simulink model "Modelisation_2_MGI_comparaison_avec_Clavel"  (R2015a)
settings: Solver=ode45  StartTime=0.0  StopTime=3  MaxStep=0.001  RelTol=1e-3
undefined symbols (not defined in the file or in its folder): sfun3d
settings Model: Creator=user  LastModifiedBy=user

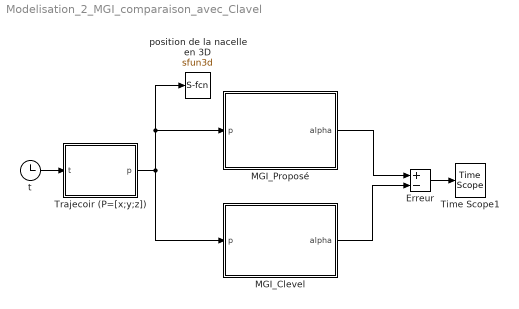
== system Modelisation_2_MGI_comparaison_avec_Clavel ==
  Erreur : Sum  Inputs=+-
  MGI_Clevel : MATLAB Function  TreatAsAtomicUnit=on
  MGI_Proposé : MATLAB Function  TreatAsAtomicUnit=on
  Time Scope1 : TimeScope  DefaultConfigurationName=spbscopes.TimeScopeBlockCfg
  Trajecoir (P=[x;y;z]) : MATLAB Function  TreatAsAtomicUnit=on
  "position de la nacelle en 3D " : S-Function  LoadFcn=sfun3d([],[],[],'LoadBlock')  StartFcn=sfun3d([],[],[],'Start')  StopFcn=sfun3d([],[],[],'Stop')  FunctionName=sfun3d  Parameters=ax,T,np,cp,gd,ls,mk  mask(3D Graph){np=1, ax=[-1 1 -1 1 -2 0]*0.3, cp=[3 2 1], gd=on, ls=-, mk=o, T=0.001}
      mask prompts: np "Number of point (lines)"; ax "[xmin xmax  ymin ymax zmin zmax]"; cp "Camera position (use [0 0 1] for 2D XY view)"; gd "Grid (on|off)"; ls "LineStyle"; mk "Marker"; T "Sampling Time"
      mask help:
      | This block plots the position of several points in the XYZ space. The input contains the coordinates of all the points (x1,y1,z1,x2,y2,z2,...).
      | The number of points (lines), the XYZ ranges, camera position, grid, linestyle, marker and sampling time, can be set as mask parameters.
      settings: CopyFcn=sfun3d([],[],[],'CopyBlock')  DeleteFcn=sfun3d([],[],[],'DeleteBlock')  NameChangeFcn=sfun3d([],[],[],'NameChange')
      mask Help:
      | This block plots the position of several points in the XYZ space. The input contains the coordinates of all the points (x1,y1,z1,x2,y2,z2,...).
      | The number of points (lines), the XYZ ranges, camera position, grid, linestyle, marker and sampling time, can be set as mask parameters.
      mask TypeOptions ls: - | -- | : | -. | none
      mask TypeOptions mk: none | . | + | o | * | x | square | diamond | v | ^ | > | < | pentagram | hexagram
      mask Display: plot([.05 .95 .95 .05 .05],[.45 .45 .95 .95 .45], 0.5+cos(0:0.1:2*pi)*0.3,0.7+sin(0:0.1:2*pi)*0.2)
  t : Clock
  wires:
  t/1 -> Trajecoir (P=[x;y;z])/1(t)
  Erreur/1 -> Time Scope1/1
  Trajecoir (P=[x;y;z])/1(p) -> "position de la nacelle en 3D "/1, MGI_Proposé/1(p), MGI_Clevel/1(p)
  MGI_Proposé/1(alpha) -> Erreur/1
  MGI_Clevel/1(alpha) -> Erreur/2

== matlab function Modelisation_2_MGI_comparaison_avec_Clavel/MGI_Proposé ==
  data: p input; alpha output
function alpha = MGI(p)

l1 = 0.19992; 
l2 = 0.334; 
r = 0.126; 
phi2 = 2*pi/3;
phi3 = 4*pi/3;

%% projection de P sur Ri
A2=[cos(phi2) sin(phi2) 0
    -sin(phi2) cos(phi2) 0
    0            0      1 ]; 
A3=[cos(phi3) sin(phi3) 0
    -sin(phi3) cos(phi3) 0
    0            0      1 ];
p2=A2*p; p3=A3*p ;

x1=p(1); y1=p(2) ; z1=p(3) ; %% p1=p
x2=p2(1); y2=p2(2) ; z2=p2(3) ;
x3=p3(1); y3=p3(2) ; z3=p3(3) ;

%% Calcule de ABi et ei :
AB1=sqrt(z1^2+(x1-r)^2);
e1=sqrt(l2^2-y1^2); 
AB2=sqrt(z2^2+(x2-r)^2);
e2=sqrt(l2^2-y2^2);
AB3=sqrt(z3^2+(x3-r)^2);
e3=sqrt(l2^2-y3^2);

%% calcul de alpha1
beta1=atan2(-z1,x1-r);
gama1=acos((AB1^2 + l1^2 - e1^2)/(2*l1*AB1));
alpha11=beta1-gama1; 
alpha12=beta1+gama1; 

%% calcul de alpha2
beta2=atan2(-z2,x2-r);
gama2=acos((AB2^2 + l1^2 - e2^2)/(2*l1*AB2));
alpha21=beta2-gama2; 
alpha22=beta2+gama2; 

%% calcul de alpha3
beta3=atan2(-z3,x3-r);
gama3=acos((AB3^2 + l1^2 - e3^2)/(2*l1*AB3));
alpha31=beta3-gama3; 
alpha32=beta3+gama3; 

%% Premiere Solution, Deuxieme Solution :
alpha=[alpha11;alpha21;alpha31];
% solution2=[alpha12,alpha22,alpha32];

== matlab function Modelisation_2_MGI_comparaison_avec_Clavel/MGI_Clevel ==
  data: p input; alpha output
function alpha = MGI(p)

x=p(1); y=p(2) ; z=p(3);

%% lesconstantes
l1 = 0.19992; 
l2 = 0.334; 
r = 0.126; 
phi1 = 0 ;
phi2 = 2*pi/3;
phi3 = 4*pi/3;

%% Clacule de Alpha_i :
 A = -2*l1*z*[1; 1; 1];

 B = [2*r*l1 - 2*l1*x*cos(phi1) - 2*l1*y*sin(phi1);
      2*r*l1 - 2*l1*x*cos(phi2) - 2*l1*y*sin(phi2);
      2*r*l1 - 2*l1*x*cos(phi3) - 2*l1*y*sin(phi3)];

 C = [l2^2 - l1^2 - r^2 + 2*r*y*sin(phi1) - z^2 - y^2 - x^2 + 2*r*x*cos(phi1);
l2^2 - l1^2 - r^2 + 2*r*y*sin(phi2) - z^2 - y^2 - x^2 + 2*r*x*cos(phi2);
l2^2 - l1^2 - r^2 + 2*r*y*sin(phi3) - z^2 - y^2 - x^2 + 2*r*x*cos(phi3)];

alpha1 = 2*atan((-A(1) + sqrt((A(1)^2 + B(1)^2 - C(1)^2)))/(B(1) + C(1)));
alpha2 = 2*atan((-A(2) + sqrt((A(2)^2 + B(2)^2 - C(2)^2)))/(B(2) + C(2)));
alpha3 = 2*atan((-A(3) + sqrt((A(3)^2 + B(3)^2 - C(3)^2)))/(B(3) + C(3)));

alpha=[alpha1;alpha2;alpha3];

== matlab function Modelisation_2_MGI_comparaison_avec_Clavel/Trajecoir (P=[x;y;z]) ==
  data: t input; p output
function p = fcn(t)
 
f = 3; 
R=0.25;
x=R*cos(f*t) ; y=R*sin(f*t) ; z=-0.35;

p=[x ; y ; z];
